simulink model "observer"  (R2020b)
settings: Solver=VariableStepAuto  StartTime=0.0  StopTime=10.0  RelTol=1e-3
undefined symbols (not defined in the file or in its folder): sim_Aobs, sim_Bobs, sim_Cobs, sim_d0obs, sim_nu, sim_nx, sim_ny, sim_TsObs, sim_x0obs
settings Model: Creator=Alessandro  LastModifiedBy=Alessandro

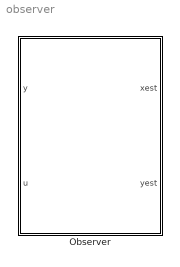
== system observer ==
  Observer : Subsystem

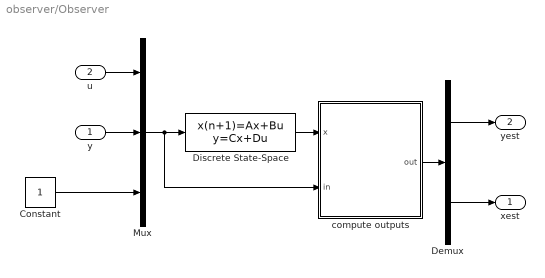
== system observer/Observer ==
  y : Inport
  u : Inport  Port=2
  Constant : Constant
  Demux : Demux  Outputs=[sim_ny sim_nx]
  Discrete State-Space : DiscreteStateSpace  A=sim_Aobs  B=sim_Bobs  C=eye(size(sim_Aobs))  D=zeros(size(sim_Aobs,1),size(sim_Bobs,2))  InitialCondition=[sim_x0obs; sim_d0obs]  SampleTime=sim_TsObs
  Mux : Mux  Inputs=3
  compute outputs : Subsystem
  xest : Outport
  yest : Outport  Port=2
  wires:
  Mux/1 -> compute outputs/2(in), Discrete State-Space/1
  Discrete State-Space/1 -> compute outputs/1(x)
  Constant/1 -> Mux/3
  u/1 -> Mux/1
  y/1 -> Mux/2
  Demux/1 -> yest/1
  Demux/2 -> xest/1
  compute outputs/1(out) -> Demux/1

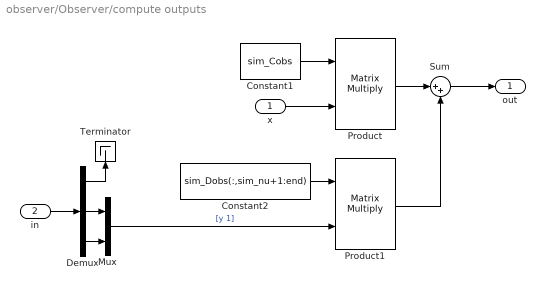
== system observer/Observer/compute outputs ==
  x : Inport
  in : Inport  Port=2
  Constant1 : Constant  Value=sim_Cobs
  Constant2 : Constant  Value=sim_Dobs(:,sim_nu+1:end)
  Demux : Demux  Outputs=[sim_nu sim_ny 1]
  Mux : Mux  Inputs=2
  Product : Product  Multiplication=Matrix(*)  SampleTime=sim_TsObs
  Product1 : Product  Multiplication=Matrix(*)  SampleTime=sim_TsObs
  Sum : Sum  Inputs=|++
  Terminator : Terminator
  out : Outport
  wires:
  in/1 -> Demux/1
  Sum/1 -> out/1
  Constant1/1 -> Product/1
  x/1 -> Product/2
  Demux/2 -> Mux/1
  Demux/3 -> Mux/2
  Demux/1 -> Terminator/1
  Mux/1 -> Product1/2  "[y 1]"
  Constant2/1 -> Product1/1
  Product/1 -> Sum/1
  Product1/1 -> Sum/2
